simulink model "ar06_ident_v00"  (R2020a)
settings: Solver=ode45  StartTime=0.0  StopTime=100  FixedStep=SIMstepSize  MaxStep=0.02  RelTol=1e-3  EnableMultiTasking=on
values from neighbouring files (symbols this model uses):
  data_Ts = 0.02    [ar06_runme_ident_v00.m]
  ok_u_PB1 = 20    [ar06_runme_ident_v00.m]
  u_PB1 = 112    [ar06_runme_ident_v00.m]
  u_PB2 = 212    [ar06_runme_ident_v00.m]
settings Model: Creator=MT  LastModifiedBy=MT
settings DataIOCC: LimitDataPoints=on  SaveFormat=Array  SignalLoggingSaveFormat=ModelDataLogs  SaveOutput=off  SignalLogging=off  DSMLogging=off  SaveTime=off  ReturnWorkspaceOutputs=off
settings OptimizationCC: ExpressionDepthLimit=2147483647  LifeSpan=inf
settings DebuggingCC: UnderspecifiedInitializationDetection=Classic  MergeDetectMultiDrivingBlocksExec=none  SolverPrmCheckMsg=warning  FcnCallInpInsideContextMsg=warning  StateNameClashWarn=warning  SFUnexpectedBacktrackingDiag=warning  SFNoUnconditionalDefaultTransitionDiag=warning  SFExecutionAtInitializationDiag=none  ArithmeticOperatorsInVariantConditions=warning
settings HardwareCC: ProdBitPerPointer=32  ProdBitPerSizeT=32  ProdBitPerPtrDiffT=32  ProdLargestAtomicFloat=None  ProdIntDivRoundTo=Undefined  ProdEndianess=Unspecified  ProdWordSize=32  ProdHWDeviceType=32-bit Generic
settings ModelReferenceCC: PropagateSignalLabelsOutOfModel=off
settings SFSimCC: SimUseLocalCustomCode=off  CustomCodeUndefinedFunction=UseInterfaceOnly
settings RTWCC: RTWUseLocalCustomCode=off
settings CodeAppCC: StateflowObjectComments=on
settings GRTTargetCC: TargetLangStandard=C89/C90 (ANSI)  CombineOutputUpdateFcns=off  GRTInterface=on
settings ConfigComp: CovMetricSettings=dw  CovHtmlReporting=on  CovSaveCumulativeToWorkspaceVar=on  CovSaveSingleToWorkspaceVar=on  CovExternalEMLEnable=off

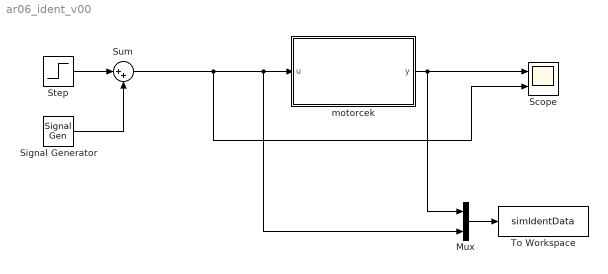
== system ar06_ident_v00 ==
  Mux : Mux  Inputs=2
  Scope : Scope  NumInputPorts=2
  Signal Generator : SignalGenerator  WaveForm=square  Amplitude=-ok_u_PB1  Frequency=1/10
  Step : Step  Time=50  Before=u_PB1  After=u_PB2  SampleTime=0
  Sum : Sum  Inputs=|++
  To Workspace : ToWorkspace  VariableName=simIdentData  SaveFormat=Timeseries  SampleTime=data_Ts
  motorcek : Subsystem
  wires:
  Step/1 -> Sum/1
  Sum/1 -> Scope/2, Mux/2, motorcek/1(u)
  Signal Generator/1 -> Sum/2
  motorcek/1(y) -> Mux/1, Scope/1
  Mux/1 -> To Workspace/1

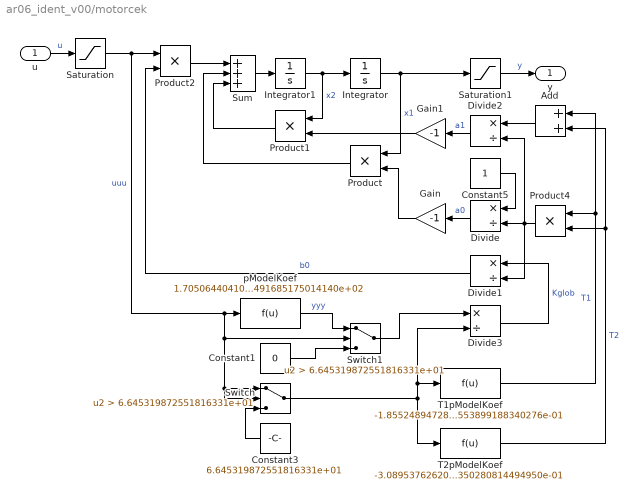
== system ar06_ident_v00/motorcek ==
  u : Inport
  Add : Sum
  Constant1 : Constant  Value=0
  Constant3 : Constant  Value=6.645319872551816331e+01
  Constant5 : Constant
  Divide{,1..3} (4 alike) : Product  Inputs=*/
  Gain : Gain  Gain=-1
  Gain1 : Gain  Gain=-1
  Integrator : Integrator
  Integrator1 : Integrator
  Product{,1..2,4} (4 alike) : Product
  Saturation : Saturate  UpperLimit=255  LowerLimit=0
  Saturation1 : Saturate  UpperLimit=1024  LowerLimit=0
  Sum : Sum  Inputs=+++
  Switch : Switch  Criteria=u2 > Threshold  Threshold=6.645319872551816331e+01
  Switch1 : Switch  Criteria=u2 > Threshold  Threshold=6.645319872551816331e+01
  T1pModelKoef : Fcn  Expr=|
      | -1.855248947282966930e-09  * u^4
      |  + 1.216542413400006364e-06  * u^3
      | -2.942513981895642059e-04 * u^2 +
      | 3.083598699517012265e-02 * u^1
      | -8.397553899188340276e-01
  T2pModelKoef : Fcn  Expr=|
      | -3.089537626202679905e-10 * u^4 +
      | 1.975259557204926176e-07 * u^3
      | -4.612506335382605391e-05 * u^2 +
      | 4.634039731493492902e-03 * u^1
      | -1.154350280814494950e-01
  pModelKoef : Fcn  Expr=|
      | 1.705064404108231154e-06  * u^4 
      | -1.154349138670292740e-03  * u^3 +
      | 2.686827024208264802e-01  * u^2
      | -2.032585984915332844e+01 * u^1+
      | 4.730491685175014140e+02
  y : Outport
  wires:
  Gain/1 -> Product/2
  Saturation/1 -> Product2/1, Switch/2, Switch/1, Switch1/2, pModelKoef/1  "uuu"
  Product1/1 -> Sum/3
  Sum/1 -> Integrator1/1
  Product4/1 -> Divide1/2, Divide2/2, Divide/2
  Constant5/1 -> Divide/1
  T1pModelKoef/1 -> Add/1, Product4/1  "T1"
  Integrator/1 -> Saturation1/1, Product/1  "x1"
  Divide1/1 -> Product2/2  "b0"
  T2pModelKoef/1 -> Add/2, Product4/2  "T2"
  Integrator1/1 -> Integrator/1, Product1/1  "x2"
  Product/1 -> Sum/2
  Gain1/1 -> Product1/2
  Divide/1 -> Gain/1  "a0"
  Product2/1 -> Sum/1
  Switch/1 -> T2pModelKoef/1, Divide3/2, T1pModelKoef/1
  Constant3/1 -> Switch/3
  Divide2/1 -> Gain1/1  "a1"
  Add/1 -> Divide2/1
  Saturation1/1 -> y/1  "y"
  u/1 -> Saturation/1  "u"
  Constant1/1 -> Switch1/3
  pModelKoef/1 -> Switch1/1  "yyy"
  Switch1/1 -> Divide3/1
  Divide3/1 -> Divide1/1  "Kglob"
